simulink model "five_bar_model"  (R2018a)
settings: Solver=ode4  StartTime=0.0  StopTime=10  FixedStep=0.0001  RelTol=1e-3
values from neighbouring files (symbols this model uses):
  g = 9.80665    [ddyn5.m]    (also in idyn5.m = -9.80665; test_dynamics.m = -9.80665; test_model.m)
  q = [NaN; NaN; NaN; NaN; NaN]    [fkine5.m]    (also in ikine5.m = [q11;q12;q13;q21;q22])
  qa = [q11;q21]    [ikine5.m]    (also in model_parameters_v_1.m = ones(length(q_(1,:)),1) * 50; test_model.m = [q(1,:);q(4,:)])
  t0r = J * qda    [ffirstkine5.m]    (also in test_dynamics.m = [0;0]; test_kinematics.m = [1;1]; test_model.m = p)
  t0rd = (J * qdda+ at)    [fsecondkine5.m]    (also in test_dynamics.m = [0;0]; test_kinematics.m = [-1;1]; test_model.m = p)
  x0 = p(1,1)    [model_parameters_v_1.m]    (also in test_model.m)
  y0 = p(2,1)    [model_parameters_v_1.m]    (also in test_model.m = p(1,2))
undefined symbols (not defined in the file or in its folder): X, Y, Z
libraries: sm_lib x23, simulink x10, nesl_utility x9, fl_lib x2
(part 2 of 2)

== matlab function five_bar_model/inverse first kinematics ==
  data: t0r input; qd output; p input double size=2; q input; qda output; qdu output; Ar output; B output; J output; Jinv output; Jt output; Jta output; Jtd output; Psit output
function [qd,qda,qdu,Ar,B,J,Jinv,Jt,Jta,Jtd,Psit] = ifirstkine5(t0r,p,q)
% This function implement the firs-order inverse kinematics model of a five bar robot
% @param t0r: twist end-effector vector 2X1
% @param p: end-effector coordinate vector 2X1
% @param q: joint positions vector 5x1
% @return qd: velocity joints vector 5x1
% @return qda: active velocity joints vector 2X1
% @return qdu: underactuated velocity joints vector 3X1
% @return Ar: matrix 2x2 relates the n dof independent coordinates of the platform twist 0 t r to the actuated joints q̇ a
% @return B: matrix 2x2 for computation of the dynamic model of the PKM
% @return J: kinematic Jacobian matrix of the PKM
% @return Jinv: inverse kinematic Jacobian matrix of the PKM
% @return Jt: crucial for computation of the dynamic model of the PKM.
% @return Jta: crucial for computation of the dynamic model of the PKM.
% @return Jtd: crucial for computation of the dynamic model of the PKM.
% @return Psit: matrix 2X6

    l = 0.205;
    d1 = [-0.125, l, l];
    d2 = [0.125, l, l];
    q1 = q(1:3);
    q2 = q(4:5);
    Phi = sum(q1);
    x = p(1);
    y = p(2);

    B = [ -d1(2)*sin(q1(2)), 0;
          0, -d2(2)*sin(q2(2))];


    Ar = [cos(q1(1) + q1(2)), sin(q1(1) + q1(2));
          cos(q2(1) + q2(2)), sin(q2(1) + q2(2))];
    % forward model
    J = -B / Ar;
    % t0r = J * qda;
    % t0r =[ -(d1(2)*qd11*sin(q2(1) + q2(2))*sin(q1(2)) - ...
    %                 d2(2)*qd21*sin(q1(1) + q1(2))*sin(q2(2)))/sin(q1(1) + q1(2) - q2(1) - q2(2));
    %         (d1(2)*qd11*cos(q2(1) + q2(2))*sin(q1(2)) - ...
    %                 d2(2)*qd21*cos(q1(1) + q1(2))*sin(q2(2)))/sin(q1(1) + q1(2) - q2(1) - q2(2))];

    Jinv = -Ar / B;
    qda = Jinv * t0r;
    % qda = [(xd*cos(q1(1) + q1(2)) + yd*sin(q1(1) + q1(2)))/(d1(2)*sin(q1(2)));
    %        (xd*cos(q2(1) + q2(2)) + yd*sin(q2(1) + q2(2)))/(d2(2)*sin(q2(2)))];


    ay = cos(Phi)^2 / (x - d2(2)*cos(q2(1)) - d2(1));
    ax = - ((y-d2(2)*sin(q2(1)))*cos(Phi)^2) / (x - d2(2)*cos(q2(1)) - d2(1))^2;
    aq = -(d2(2) * ((x-d2(1))*cos(q2(1))+y*sin(q2(1))-d2(2))*cos(Phi)^2) / (x - d2(2)*cos(q2(1)) - d2(1))^2;

    Psit = [1                     0
            0                     1
            0                     0
            0                     0
            0                     0
            (ax+aq*Jinv(2,1)) (ay+aq*Jinv(2,2))];

    Jt = [-sin(q1(1) + q1(2)),cos(q1(1) + q1(2));
            (ax + aq*Jinv(2,1)), (ay + aq*Jinv(2,2));
            -sin(q2(1) + q2(2)),cos(q2(1) + q2(2))];


    Jta = [ d1(3) + d1(2)*cos(q1(2)), 0;
            1,                0;
            0,      d2(3) + d2(2)*cos(q2(2))];

    Jtd = [ d1(3), 0,   0;
            1,   1,   0;
            0,   0, d2(3)];

    qdu = inv(Jtd)*(Jt * t0r - Jta * qda); 
    qd = [qda(1);qdu(1);qdu(2);qda(2);qdu(3)];

== matlab function five_bar_model/inverse secod kinematics ==
  data: t0rd input; qdd output; t0r input; p input double size=2; q input; qd input; Ar input; B input; Jinv input; Jt input; Jta input; Jtd input; Psit input; qdda output; qddu output; Psit1 output; Psit2 output; atp output; ad output
function [qdd,qdda,qddu,Psit1,Psit2,atp,ad] = isecondkine5(t0rd,t0r,p,q,qd,Ar,B,Jinv,Jt,Jta,Jtd,Psit)
% This function implement the second-order inverse kinematics model of a five bar robot
% @param t0rd: derivate twist end-effector vector 2X1
% @param t0r: twist end-effector vector 2X1
% @param p: end-effector coordinate vector 2X1
% @param q: joint positions vector 5x1
% @param qd: velocity joints vector 5x1
% @param Ar: matrix 2x2 for computation of the dynamic model of the PKM
% @param B: matrix 2x2 for computation of the dynamic model of the PKM
% @param Jinv: inverse kinematic Jacobian matrix of the PKM
% @param Jt: crucial for computation of the dynamic model of the PKM.
% @param Jta: crucial for computation of the dynamic model of the PKM.
% @param Jtd: crucial for computation of the dynamic model of the PKM.
% @return qdd: acceleration joint vector 5x1
% @return qdda: active acceleration joints vector 2X1
% @return qddu: underactuated acceleration joints vector 3X1
% @return Psit1: matrix 2x6
% @return Psit2: matrix 1x6
% @return atp: acceleration using for dynamics
% @return ad: acceleration using for dynamics

    l = 0.205;
    d1 = [-0.125, l, l];
    d2 = [0.125, l, l];
    q1 = q(1:3);
    q2 = q(4:5);
    qd1 = qd(1:3);
    qd2 = qd(4:5);
    Phi = sum(q1);
    Phid = sum(qd1);
    x = p(1);
    y = p(2);
    xd = t0r(1);
    yd = t0r(2);

    wr1 = [cos(q1(1)+q1(2)); sin(q1(1)+q1(2)); 0; 0; 0; 0];
    wr2 = [cos(q2(1)+q2(2)); sin(q2(1)+q2(2)); 0; 0; 0; 0];

    b01a_ = [-d1(2)*qd1(1)*cos(q1(1)) - d1(3)*cos(q1(1)+q1(2))*(qd1(1)+qd1(2));
             -d1(2)*qd1(1)*sin(q1(1)) - d1(3)*sin(q1(1)+q1(2))*(qd1(1)+qd1(2));
             zeros(4,1)];
    b01b_ = [-d1(3)*cos(q1(1)+q1(2));
             -d1(3)*sin(q1(1)+q1(2));
             zeros(4,1)];
    b0p1 = b01a_ * qd1(1) + b01b_ * qd1(2)*(qd1(1)+qd1(2));

    b02a_ = [-d2(2)*qd2(1)*cos(q2(1)) - d2(3)*cos(q2(1)+q2(2))*(qd2(1)+qd2(2));
             -d2(2)*qd2(1)*sin(q2(1)) - d2(3)*sin(q2(1)+q2(2))*(qd2(1)+qd2(2));
             zeros(4,1)];
    b02b_ = [-d2(3)*cos(q2(1)+q2(2));
             -d2(3)*sin(q2(1)+q2(2));
             zeros(4,1)];
    b0p2 = b02a_ * qd2(1) + b02b_ * qd2(2)*(qd2(1)+qd2(2));

    b0p = [(wr1'*b0p1); (wr2'*b0p2)];

    aqq = inv(B) * b0p;
    qdda = (Jinv * t0rd + aqq);

    % Aceleracion pasiva

    ayd = (Phid*sin(2*Phi))/(d2(1) - x + d2(2)*cos(q2(1))) - (cos(Phi)^2*(xd + d2(2)*qd2(1)*sin(q2(1))))/(d2(1) - x + d2(2)*cos(q2(1)))^2;

    axd = (Phid*sin(2*Phi)*(y - d2(2)*sin(q2(1))))/(d2(1) - x + d2(2)*cos(q2(1)))^2 ...
        - (cos(Phi)^2*(yd - d2(2)*qd2(1)*cos(q2(1))))/(d2(1) - x + d2(2)*cos(q2(1)))^2 ...
        - (2*cos(Phi)^2*(xd + d2(2)*qd2(1)*sin(q2(1)))*(y - d2(2)*sin(q2(1))))/(d2(1) - x + d2(2)*cos(q2(1)))^3;

    aqd = (2*d2(2)*cos(Phi)^2*(xd + d2(2)*qd2(1)*sin(q2(1)))*(d2(2) - sin(q2(1))*y + cos(q2(1))*(d2(1) - x)))...
        /(d2(1) - x + d2(2)*cos(q2(1)))^3 ...
        - (d2(2)*cos(Phi)^2*(xd*cos(q2(1)) + yd*sin(q2(1)) + qd2(1)*cos(q2(1))*y + qd2(1)*sin(q2(1))*(d2(1) - x)))...
        /(d2(1) - x + d2(2)*cos(q2(1)))^2 ...
        - (2*Phid*d2(2)*cos(Phi)*sin(Phi)*(d2(2) - sin(q2(1))*y + cos(q2(1))*(d2(1) - x)))...
        /(d2(1) - x + d2(2)*cos(q2(1)))^2;

    j21_invd = -(sin(q2(1) + q2(2))*(qd2(1) + qd2(2)))/(d2(2)*sin(q2(2))) ...
               -(qd2(2)*cos(q2(1) + q2(2))*cos(q2(2)))/(d2(2)*sin(q2(2))^2);

    j22_invd = -(qd2(2)*sin(q2(1) + q2(2))*cos(q2(2)))/(d2(2)*sin(q2(2))^2) ...
               +(cos(q2(1) + q2(2))*(qd2(1) + qd2(2)))/(d2(2)*sin(q2(2)));

    aq = -(d2(2) * ((x-d2(1))*cos(q2(1))+y*sin(q2(1))-d2(2))*cos(Phi)^2) / (x - d2(2)*cos(q2(1)) - d2(1))^2;

    psitd1 = axd + aqd*Jinv(2,1)+ aq*j21_invd;
    psitd2 = ayd + aqd*Jinv(2,2)+ aq*j22_invd;

    Psidt = [0 0; 0 0; 0 0; 0 0; 0 0; psitd1 psitd2];

    Psit1 = [-sin(q1(1)+q1(2)) cos(q1(1)+q1(2)) 0 0 0 0
             0                 0                0 0 0 1];
    Psit2 = [-sin(q2(1)+q2(2)) cos(q2(1)+q2(2)) 0 0 0 0];

    dc1 = Psit1 * (eye(6)* Psidt * t0r - b0p1);
    dc2 = Psit2 * (eye(6)* Psidt * t0r - b0p2);
    dc = [dc1;
          dc2];

    qddu =  inv(Jtd)*(Jt*t0rd - Jta*qdda + dc);

    qdd = [qdda(1);qddu(1);qddu(2);qdda(2);qddu(3)];

    at = inv(Ar) * b0p;
    atp = Psit * at + Psidt * t0r;% using for dynamics
    ad = inv(Jtd) * (dc + Jt*at); % For dynamics

== matlab function five_bar_model/forward kinematics ==
  data: qa_act input; p_act output double size=2; q_act output; p_ant input; q_ant input
function [p_act, q_act]  = fkine5(qa_act, p_ant, q_ant)
% This function implement the forward kinematic model of a five bar robot
% @parm q: joint positions vector 5x1
% @return p: p end-effector coordinate vector 2X1
    l = 0.205;
    d1 = [-0.125, l, l];
    d2 = [0.125, l, l];
    q1 = qa_act(1);
    q2 = qa_act(2);

    A12 = [d1(2)*cos(q1(1))+d1(1); d1(2)*sin(q1(1))];
    A22 = [d2(2)*cos(q2(1))+d2(1); d2(2)*sin(q2(1))];
    s = sqrt(sum((A22-A12).^2));
    if s <= 2*l
        a1 = - 2*d1(1) - 2*d1(2)*cos(q1(1));
        a2 = - 2*d2(1) - 2*d2(2)*cos(q2(1));
        b1 = - 2*sin(q1(1))*d1(2);
        b2 = - 2*sin(q2(1))*d2(2);
        c1 = d1(1)^2 + 2*cos(q1(1))*d1(1)*d1(2) + d1(2)^2 - d1(3)^2;
        c2 = d2(1)^2 + 2*cos(q2(1))*d2(1)*d2(2) + d2(2)^2 - d2(3)^2;

        if b1 ~= b2
            a = a2 - a1;
            b = b2 - b1;
            c = c2 - c1;
            e1 = - a / b;
            e2 = - c / b;
            f1 = 1 + e1^2;
            f2 = 2 * e1 * e2 + a1 + b1 * e1;
            f3 = e2^2 + b1 * e2 + c1;

            x = (-f2 - sqrt(f2^2 - 4 * f1 * f3)) / (2 * f1);
            y = e1 * x + e2;

            A13=[A12(1)-x;A12(2)-y];
            A23=[A22(1)-x;A22(2)-y];
            if  A13(1)*A23(2)-A23(1)*A13(2) <= 0
                x = (-f2 + sqrt(f2^2 - 4 * f1 * f3)) / (2 * f1);
                y = e1 * x + e2;
            end
        else
            x = - (c2 - c1) / (a2 - a1);
            y = (-b1 + (b1^2 - 4 * (x^2 + a1 * x + c1))^(1/2)) / 2;

            A13=[A12(1)-x;A12(2)-y];
            A23=[A22(1)-x;A22(2)-y];
            if  A13(1)*A23(2)-A23(1)*A13(2) <= 0
                y = (-b1 - (b1^2 - 4 * (x^2 + a1 * x + c1))^(1/2)) / 2;
            end
        end

        % for q12 and q22 from a12/a11 and a22/a21
        q12 = atan2(y-d1(2)*sin(q1(1)), x-d1(1)-d1(2)*cos(q1(1))) - q1(1);
        q22 = atan2(y-d2(2)*sin(q2(1)), x-d2(1)-d2(2)*cos(q2(1))) - q2(1);
        q13 = q2(1) + q22 - q1(1) - q12;
        q_act = [q1(1); q12; q13; q2(1); q22];
        p_act = [x;y];
    else
        p_act = p_ant;
        q_act = q_ant;
%         x = p(1);
%         y = p(2);
%         q1(1) = q_ant(1);
%         q2(1) = q_ant(2);
%         q12 = atan2(y-d1(2)*sin(q1(1)), x-d1(1)-d1(2)*cos(q1(1))) - q1(1);
%         q22 = atan2(y-d2(2)*sin(q2(1)), x-d2(1)-d2(2)*cos(q2(1))) - q2(1);
%         q13 = q2(1) + q22 - q1(1) - q12;
%         q_ = [q1(1); q12; q13; q2(1); q22];
        
    end
